simulink model "Problem2"  (R2020b)
settings: Solver=VariableStepAuto  StartTime=0.0  StopTime=10.0  RelTol=1e-3
model workspace (MAT data in the model file):
  Fn = Simulink.Parameter
  Fn.Value = [0  0; 1  0.8; 2  1.6; 3  1.6; 4  1.6; 5  1.6; 6  0.8; 7  0; 8  0; 9  0; 10  0]
  Fn.DataType = 'auto'
  Fn.Dimensions = [11 2]
  R = Simulink.Parameter
  R.Value = 1
  R.DataType = 'auto'
  R.Dimensions = [1 1]
  Sig = Simulink.Signal
  Sig.DataType = 'auto'
  Sig.Dimensions = -1
  Sig.DimensionsMode = 'auto'
  Sig.Complexity = 'auto'
  Sig.SampleTime = -1
  Sig.SamplingMode = 'auto'
  Tin = Simulink.Parameter
  Tin.Value = [1  2; 2  2; 3  2; 4  2; 5  2; 6  0; 7  0; 8  0; 9  0; 10  0]
  Tin.DataType = 'auto'
  Tin.Dimensions = [10 2]
  be = Simulink.Parameter
  be.Value = 2
  be.DataType = 'auto'
  be.Dimensions = [1 1]
  bv = Simulink.Parameter
  bv.Value = 1
  bv.DataType = 'auto'
  bv.Dimensions = [1 1]
  f1 = Simulink.Parameter
  f1.Value = [1; 6; 11; 16; 21; 26; 31; 36; 41; 46; 51]
  f1.DataType = 'auto'
  f1.Dimensions = [11 1]
  le = Simulink.Parameter
  le.Value = 1
  le.DataType = 'auto'
  le.Dimensions = [1 1]
  lv = Simulink.Parameter
  lv.Value = 5
  lv.DataType = 'auto'
  lv.Dimensions = [1 1]
  muk = Simulink.Parameter
  muk.Value = 1
  muk.DataType = 'auto'
  muk.Dimensions = [1 1]
  mus = Simulink.Parameter
  mus.Value = 1.5
  mus.DataType = 'auto'
  mus.Dimensions = [1 1]
settings Model: DataDictionary=DD.sldd  Creator=omkar  LastModifiedBy=omkar

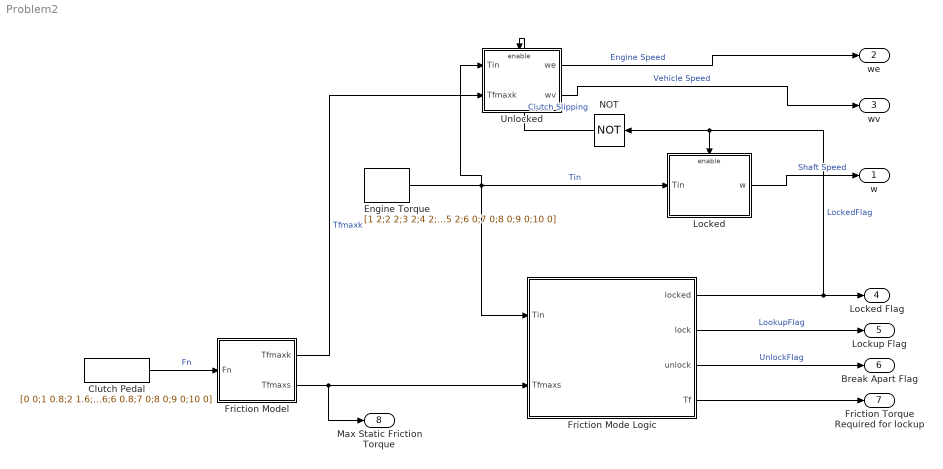
== system Problem2 ==
  Clutch Pedal : FromWorkspace  VariableName=[0 0;1 0.8;2 1.6;3 1.6;4 1.6;5 1.6;6 0.8;7 0;8 0;9 0;10 0]
  Engine Torque : FromWorkspace  VariableName=[1 2;2 2;3 2;4 2;5 2;6 0;7 0;8 0;9 0;10 0]
  Friction Mode Logic : Subsystem
  Friction Model : Subsystem
  Locked : Subsystem
  NOT : Logic  Operator=NOT  IconShape=distinctive  AllPortsSameDT=off  OutDataTypeStr=boolean
  Unlocked : Subsystem
  w : Outport
  we : Outport  Port=2
  wv : Outport  Port=3
  Locked Flag : Outport  Port=4  InitialOutput=0  VectorParamsAs1DForOutWhenUnconnected=off
  Lockup Flag : Outport  Port=5
  Break Apart Flag : Outport  Port=6
  "Friction Torque Required for lockup " : Outport  Port=7
  Max Static Friction Torque : Outport  Port=8
  wires:
  Unlocked/2(wv) -> wv/1  "Vehicle Speed"
  Friction Mode Logic/3(unlock) -> Break Apart Flag/1  "UnlockFlag"
  Unlocked/1(we) -> we/1  "Engine Speed"
  Friction Model/2(Tfmaxs) -> Friction Mode Logic/2(Tfmaxs), Max Static Friction Torque/1
  NOT/1 -> Unlocked/Enable  "Clutch Slipping"
  Engine Torque/1 -> Unlocked/1(Tin), Locked/1(Tin), Friction Mode Logic/1(Tin)  "Tin"
  Locked/1(w) -> w/1  "Shaft Speed"
  Friction Mode Logic/2(lock) -> Lockup Flag/1  "LookupFlag"
  Friction Mode Logic/1(locked) -> Locked Flag/1, Locked/Enable, NOT/1  "LockedFlag"
  Friction Model/1(Tfmaxk) -> Unlocked/2(Tfmaxk)  "Tfmaxk"
  Friction Mode Logic/4(Tf) -> "Friction Torque Required for lockup "/1
  Clutch Pedal/1 -> Friction Model/1(Fn)  "Fn"

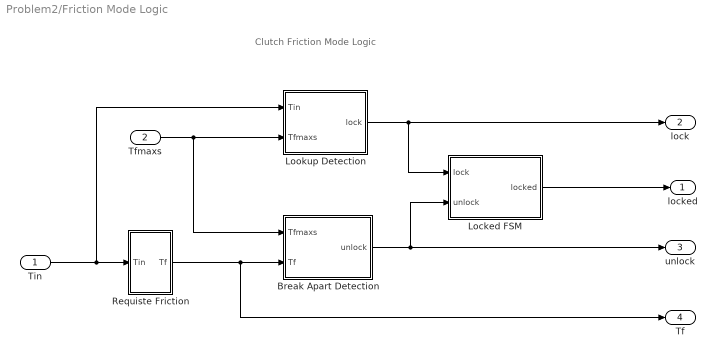
== system Problem2/Friction Mode Logic ==
  note: Clutch Friction Mode Logic
  Tin : Inport
  Tfmaxs : Inport  Port=2
  Break Apart Detection : Subsystem
  Locked FSM : Subsystem
  Lookup Detection : Subsystem
  Requiste Friction : Subsystem
  locked : Outport  InitialOutput=0  VectorParamsAs1DForOutWhenUnconnected=off
  lock : Outport  Port=2
  unlock : Outport  Port=3
  Tf : Outport  Port=4
  wires:
  Requiste Friction/1(Tf) -> Break Apart Detection/2(Tf), Tf/1
  Break Apart Detection/1(unlock) -> Locked FSM/2(unlock), unlock/1
  Lookup Detection/1(lock) -> Locked FSM/1(lock), lock/1
  Locked FSM/1(locked) -> locked/1
  Tfmaxs/1 -> Lookup Detection/2(Tfmaxs), Break Apart Detection/1(Tfmaxs)
  Tin/1 -> Requiste Friction/1(Tin), Lookup Detection/1(Tin)

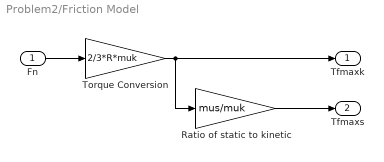
== system Problem2/Friction Model ==
  Fn : Inport
  Ratio of static to kinetic : Gain  Gain=mus/muk  SaturateOnIntegerOverflow=on  OutDataTypeStr=Inherit: Same as input  ParamDataTypeStr=Inherit: Same as input
  Torque Conversion : Gain  Gain=2/3*R*muk  SaturateOnIntegerOverflow=on  OutDataTypeStr=Inherit: Same as input  ParamDataTypeStr=Inherit: Same as input
  Tfmaxk : Outport  InitialOutput=0  VectorParamsAs1DForOutWhenUnconnected=off
  Tfmaxs : Outport  Port=2  InitialOutput=0  VectorParamsAs1DForOutWhenUnconnected=off
  wires:
  Ratio of static to kinetic/1 -> Tfmaxs/1
  Fn/1 -> Torque Conversion/1
  Torque Conversion/1 -> Ratio of static to kinetic/1, Tfmaxk/1

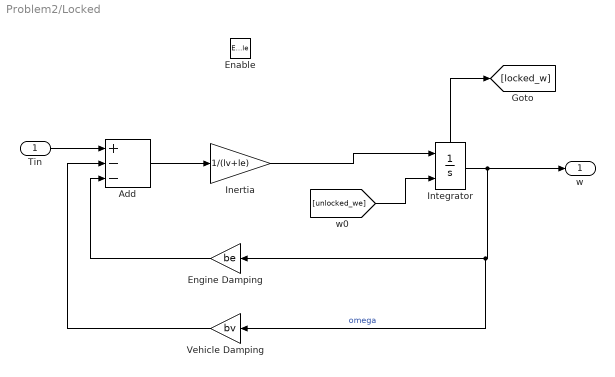
== system Problem2/Locked ==
  Tin : Inport
  Enable : EnablePort
  Add : Sum  Inputs=+--
  Engine Damping : Gain  Gain=be
  Inertia : Gain  Gain=1/(lv+le)
  Integrator : Integrator  InitialConditionSource=external  ShowStatePort=on
  Vehicle Damping : Gain  Gain=bv
  w : Outport
  wires:
  [unlocked_we] -> Integrator/2
  Integrator/1 -> Engine Damping/1, Vehicle Damping/1, w/1  "omega"
  Inertia/1 -> Integrator/1
  Vehicle Damping/1 -> Add/2
  Engine Damping/1 -> Add/3
  Integrator/State -> [locked_w]
  Add/1 -> Inertia/1
  Tin/1 -> Add/1

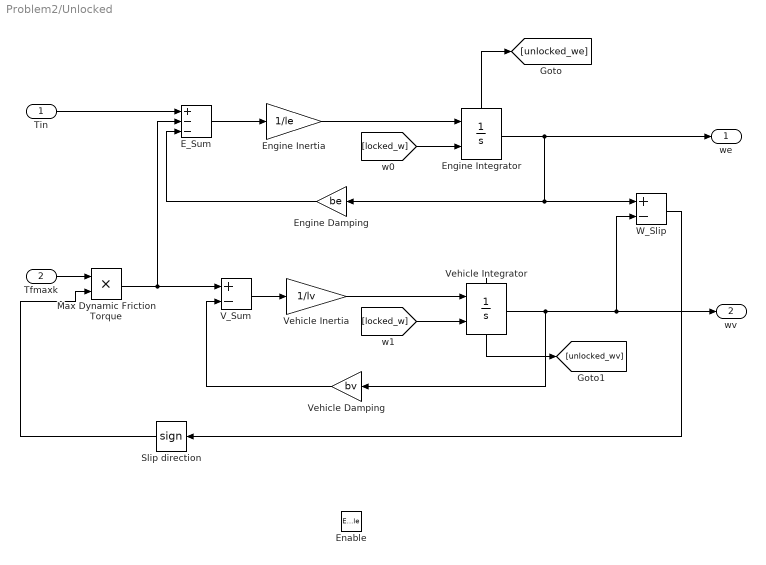
== system Problem2/Unlocked ==
  Tin : Inport
  Tfmaxk : Inport  Port=2
  Enable : EnablePort
  E_Sum : Sum  Inputs=+--
  Engine Damping : Gain  Gain=be
  Engine Inertia : Gain  Gain=1/le
  Engine Integrator : Integrator  InitialConditionSource=external  ShowStatePort=on
  Max Dynamic Friction Torque : Product
  Slip direction : Signum  ZeroCross=off
  V_Sum : Sum  Inputs=+-
  Vehicle Damping : Gain  Gain=bv
  Vehicle Inertia : Gain  Gain=1/lv
  Vehicle Integrator : Integrator  InitialConditionSource=external  ShowStatePort=on
  W_Slip : Sum  Inputs=+-
  we : Outport
  wv : Outport  Port=2
  wires:
  E_Sum/1 -> Engine Inertia/1
  W_Slip/1 -> Slip direction/1
  Engine Integrator/State -> [unlocked_we]
  [locked_w] -> Engine Integrator/2
  Vehicle Damping/1 -> V_Sum/2
  Slip direction/1 -> Max Dynamic Friction Torque/2
  Vehicle Inertia/1 -> Vehicle Integrator/1
  V_Sum/1 -> Vehicle Inertia/1
  Engine Integrator/1 -> Engine Damping/1, W_Slip/1, we/1
  Tin/1 -> E_Sum/1
  Engine Inertia/1 -> Engine Integrator/1
  Max Dynamic Friction Torque/1 -> V_Sum/1, E_Sum/2
  Engine Damping/1 -> E_Sum/3
  [locked_w] -> Vehicle Integrator/2
  Vehicle Integrator/State -> [unlocked_wv]
  Tfmaxk/1 -> Max Dynamic Friction Torque/1
  Vehicle Integrator/1 -> Vehicle Damping/1, W_Slip/2, wv/1

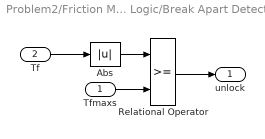
== system Problem2/Friction Mode Logic/Break Apart Detection ==
  Tfmaxs : Inport
  Tf : Inport  Port=2
  Abs : Abs  SaturateOnIntegerOverflow=on
  Relational Operator : RelationalOperator  OutDataTypeStr=boolean  RndMeth=Nearest  InputSameDT=on
  unlock : Outport  InitialOutput=0  VectorParamsAs1DForOutWhenUnconnected=off
  wires:
  Tfmaxs/1 -> Relational Operator/2
  Abs/1 -> Relational Operator/1
  Tf/1 -> Abs/1
  Relational Operator/1 -> unlock/1

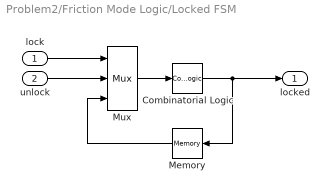
== system Problem2/Friction Mode Logic/Locked FSM ==
  lock : Inport
  unlock : Inport  Port=2
  Combinatorial Logic : CombinatorialLogic  TruthTable=[0;1;0;0;1;1;1;0]
  Memory : Memory
  Mux : Mux  Inputs=3
  locked : Outport  InitialOutput=0  VectorParamsAs1DForOutWhenUnconnected=off
  wires:
  unlock/1 -> Mux/2
  Mux/1 -> Combinatorial Logic/1
  Combinatorial Logic/1 -> Memory/1, locked/1
  Memory/1 -> Mux/3
  lock/1 -> Mux/1

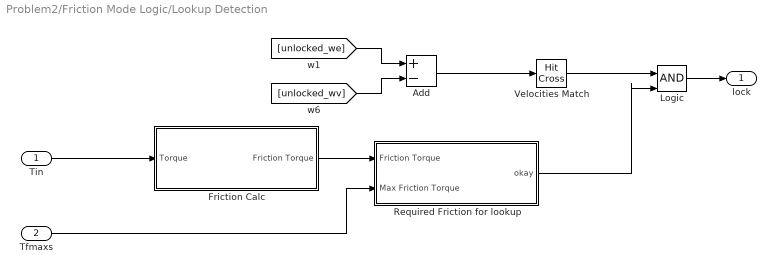
== system Problem2/Friction Mode Logic/Lookup Detection ==
  Tin : Inport
  Tfmaxs : Inport  Port=2
  Add : Sum  Inputs=+-
  Friction Calc : Subsystem
  Logic : Logic  IconShape=distinctive  OutDataTypeStr=boolean
  Required Friction for lookup : Subsystem
  Velocities Match : HitCross
  lock : Outport  InitialOutput=0  VectorParamsAs1DForOutWhenUnconnected=off
  wires:
  Required Friction for lookup/1(okay) -> Logic/2
  [unlocked_wv] -> Add/2
  Tin/1 -> Friction Calc/1(Torque)
  [unlocked_we] -> Add/1
  Friction Calc/1(Friction Torque) -> Required Friction for lookup/1(Friction Torque)
  Logic/1 -> lock/1
  Add/1 -> Velocities Match/1
  Velocities Match/1 -> Logic/1
  Tfmaxs/1 -> Required Friction for lookup/2(Max Friction Torque)

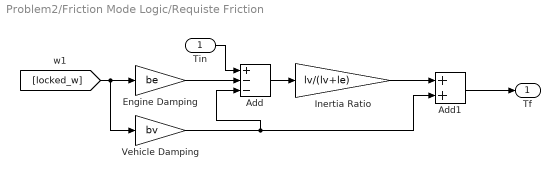
== system Problem2/Friction Mode Logic/Requiste Friction ==
  Tin : Inport
  Add : Sum  Inputs=+--
  Add1 : Sum
  Engine Damping : Gain  Gain=be  SaturateOnIntegerOverflow=on  OutDataTypeStr=Inherit: Same as input  ParamDataTypeStr=Inherit: Same as input
  Inertia Ratio : Gain  Gain=lv/(lv+le)  SaturateOnIntegerOverflow=on  OutDataTypeStr=Inherit: Same as input  ParamDataTypeStr=Inherit: Same as input
  Vehicle Damping : Gain  Gain=bv  SaturateOnIntegerOverflow=on  OutDataTypeStr=Inherit: Same as input  ParamDataTypeStr=Inherit: Same as input
  Tf : Outport  InitialOutput=0  VectorParamsAs1DForOutWhenUnconnected=off
  wires:
  Tin/1 -> Add/1
  Vehicle Damping/1 -> Add/3, Add1/2
  Engine Damping/1 -> Add/2
  Add/1 -> Inertia Ratio/1
  Inertia Ratio/1 -> Add1/1
  Add1/1 -> Tf/1
  [locked_w] -> Engine Damping/1, Vehicle Damping/1

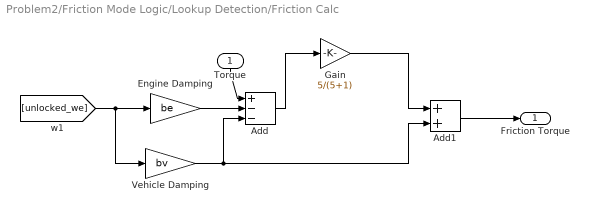
== system Problem2/Friction Mode Logic/Lookup Detection/Friction Calc ==
  Torque : Inport
  Add : Sum  Inputs=+--
  Add1 : Sum
  Engine Damping : Gain  Gain=be  SaturateOnIntegerOverflow=on  OutDataTypeStr=Inherit: Same as input  ParamDataTypeStr=Inherit: Same as input
  Gain : Gain  Gain=5/(5+1)
  Vehicle Damping : Gain  Gain=bv  SaturateOnIntegerOverflow=on  OutDataTypeStr=Inherit: Same as input  ParamDataTypeStr=Inherit: Same as input
  Friction Torque : Outport  InitialOutput=0  VectorParamsAs1DForOutWhenUnconnected=off
  wires:
  Gain/1 -> Add1/1
  Torque/1 -> Add/1
  Engine Damping/1 -> Add/2
  Add1/1 -> Friction Torque/1
  Vehicle Damping/1 -> Add/3, Add1/2
  [unlocked_we] -> Vehicle Damping/1, Engine Damping/1
  Add/1 -> Gain/1

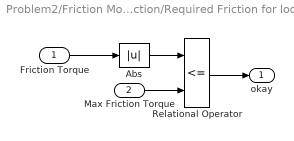
== system Problem2/Friction Mode Logic/Lookup Detection/Required Friction for lookup ==
  Friction Torque : Inport
  Max Friction Torque : Inport  Port=2
  Abs : Abs  SaturateOnIntegerOverflow=on
  Relational Operator : RelationalOperator  Operator=<=  OutDataTypeStr=boolean  RndMeth=Nearest  InputSameDT=on
  okay : Outport  InitialOutput=0  VectorParamsAs1DForOutWhenUnconnected=off
  wires:
  Max Friction Torque/1 -> Relational Operator/2
  Friction Torque/1 -> Abs/1
  Relational Operator/1 -> okay/1
  Abs/1 -> Relational Operator/1
